simulink model "carsim_interface"  (R2017a)
settings: Solver=VariableStepAuto  StartTime=0.0  StopTime=10.0  RelTol=1e-3
libraries: Solver_SF x1
settings Model: Creator=User  LastModifiedBy=User

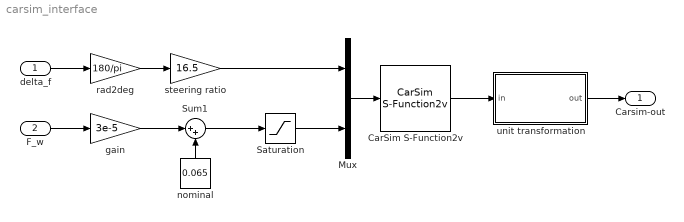
== system carsim_interface ==
  delta_f : Inport
  F_w : Inport  Port=2
  CarSim S-Function2v : Solver_SF/CarSim S-Function2v  Priority=1  VehicleCode=i_i  SIMFILE=simfile.sim
      settings: AttributesFormatString=Vehicle Code: %<VehicleCode>
  Mux : Mux  Inputs=2
  Saturation : Saturate  UpperLimit=0.2  LowerLimit=0
  Sum1 : Sum  Inputs=|++
  gain : Gain  Gain=3e-5
  nominal : Constant  Value=0.065
  rad2deg : Gain  Gain=180/pi
  steering ratio : Gain  Gain=16.5
  "unit transformation " : MATLAB Function  TreatAsAtomicUnit=on
  Carsim-out : Outport  OutDataTypeStr=Bus: DataBus
  wires:
  Sum1/1 -> Saturation/1
  F_w/1 -> gain/1
  Saturation/1 -> Mux/2
  delta_f/1 -> rad2deg/1
  rad2deg/1 -> steering ratio/1
  nominal/1 -> Sum1/2
  CarSim S-Function2v/1 -> "unit transformation "/1(in)
  Mux/1 -> CarSim S-Function2v/1
  "unit transformation "/1(out) -> Carsim-out/1
  steering ratio/1 -> Mux/1
  gain/1 -> Sum1/1

== matlab function carsim_interface/unit transformation  ==
  data: out output Bus: DataBus; in input
function out  = fcn(in)
    out.lat = in(1);
    out.long = in(2);
    out.el = 0;
    out.Yaw = deg2rad(in(3));
    out.YawRate = deg2rad(in(4));
    out.Vx = in(5)/3.6;
    out.Vy = in(6)/3.6;
    out.x_CG = in(7)/1000;
    out.y_CG = in(8)/1000;
    out.steer_L1 = deg2rad(in(9));
    out.steer_R1 = deg2rad(in(10));
    out.Alpha_L1 = deg2rad(in(11));
    out.Alpha_R1 = deg2rad(in(12));
    out.Fy_L1 = in(13);
    out.Fy_R1 = in(14);
    out.Fz_L1 = in(15);
    out.Fz_R1 = in(16);
    out.Fx  = in(17) + in(18);
